simulink library "DiscreteVariableLeadLag"  (Simulink 8.9)
settings: Solver=VariableStepAuto  StartTime=0.0  StopTime=10.0  RelTol=1e-3
undefined symbols (not defined in the file): Ts, z_d, z_n
settings Model: SuppressorTable=22 serialization::archive 11 0 6 0 0 0 0 0  Creator=hbolandhemmat  LastModifiedBy=hbolandhemmat

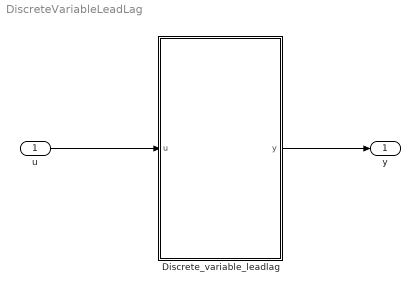
== system DiscreteVariableLeadLag ==
  u : Inport
  Discrete_variable_leadlag : Subsystem
  y : Outport
  wires:
  u/1 -> Discrete_variable_leadlag/1(u)
  Discrete_variable_leadlag/1(y) -> y/1

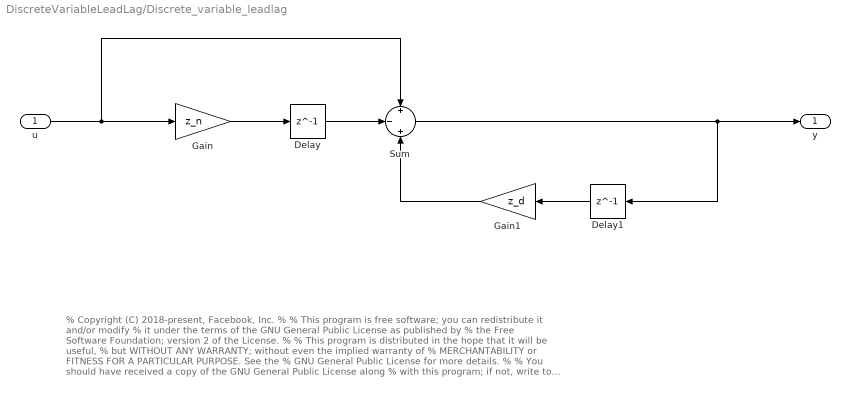
== system DiscreteVariableLeadLag/Discrete_variable_leadlag ==
  note: % Copyright (C) 2018-present, Facebook, Inc.
      | %
      | % This program is free software; you can redistribute it and/or modify
      | % it under the terms of the GNU General Public License as published by
      | % the Free Software Foundation; version 2 of the License.
      | %
      | % This program is distributed in the hope that it will be useful,
      | % but WITHOUT ANY WARRANTY; without even the implied warranty of
      | % MERCHANTABILITY or FITNESS FOR A PARTICULAR PURPOSE. See the
      | % GNU General Public License for more details.
      | %
      | % You should have received a copy of the GNU General Public License along
      | % with this program; if not, write to the Free Software Foundation, Inc.,
      | % 51 Franklin Street, Fifth Floor, Boston, MA 02110-1301 USA.
  u : Inport
  Delay : Delay  DelayLength=1  InitialCondition=0  SampleTime=Ts
  Delay1 : Delay  DelayLength=1  InitialCondition=0  SampleTime=Ts
  Gain : Gain  Gain=z_n
  Gain1 : Gain  Gain=z_d
  Sum : Sum  Inputs=+|-|+
  y : Outport
  wires:
  Delay1/1 -> Gain1/1
  u/1 -> Sum/1, Gain/1
  Delay/1 -> Sum/2
  Gain1/1 -> Sum/3
  Sum/1 -> y/1, Delay1/1
  Gain/1 -> Delay/1
